simulink model "segunda_ordem_indireta_comparacao"  (Simulink 7.9)
settings: Solver=ode45  StartTime=0.0  StopTime=10.0  RelTol=1e-3
settings Model: Creator=Danilo  LastModifiedBy=Danilo

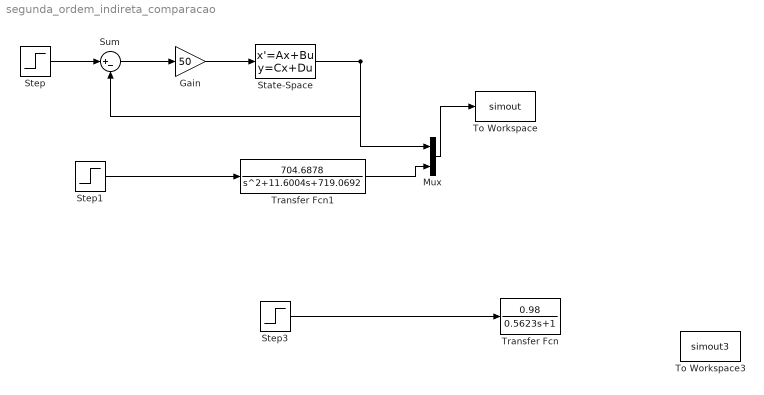
== system segunda_ordem_indireta_comparacao ==
  Gain : Gain  Gain=50
  Mux : Mux  Inputs=2
  State-Space : StateSpace  A=[-12 -16;1 0]  B=[1;0]  C=[0 16]  D=0
  Step : Step  Time=0  SampleTime=0
  Step1 : Step  Time=0  SampleTime=0
  Step3 : Step  Time=0  SampleTime=0
  Sum : Sum  Inputs=|+-
  To Workspace : ToWorkspace  VariableName=simout  SampleTime=-1
  To Workspace3 : ToWorkspace  VariableName=simout3  SampleTime=-1
  Transfer Fcn : TransferFcn  Numerator=[0.98]  Denominator=[0.5623 1]
  Transfer Fcn1 : TransferFcn  Numerator=[704.6878]  Denominator="[1  11.6004 719.0692]"
  wires:
  State-Space/1 -> Sum/2, Mux/1
  Gain/1 -> State-Space/1
  Step/1 -> Sum/1
  Sum/1 -> Gain/1
  Transfer Fcn1/1 -> Mux/2
  Step1/1 -> Transfer Fcn1/1
  Mux/1 -> To Workspace/1
  Step3/1 -> Transfer Fcn/1
